simulink model "thrust_control"  (R2017a)
settings: Solver=VariableStepAuto  StartTime=0.0  StopTime=2  MaxStep=1e-3  RelTol=1e-3
values from neighbouring files (symbols this model uses):
  A = [0 1 ... (first row only)    [system_id.m]    (also in thrust_control_data.m)
  Ad = [Ad ... (first row only)    [thrust_control_data.m]
  B = [0 ... (first row only)    [system_id.m]    (also in thrust_control_data.m)
  Bd = [zeros(n+l-1, 1) ... (first row only)    [thrust_control_data.m]
  C = [1 0]    [system_id.m]    (also in thrust_control_data.m)
  Hd = acker(Aobs', Cobs', 0.4 * ones(1, n+l+1))'    [thrust_control_data.m]
  Kd = [2000 1000]    [thrust_control_data.m]
  T = 1/30    (= 0.0333333333333)    [drone_data_process.m]    (also in thrust_control_data.m)
settings Model: Creator=sdc  LastModifiedBy=sdc

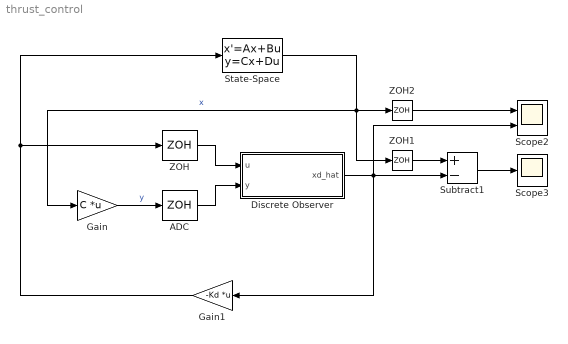
== system thrust_control ==
  ADC : ZeroOrderHold  SampleTime=T
  Discrete Observer : Subsystem
  Gain : Gain  Gain=C  Multiplication=Matrix(K*u)
  Gain1 : Gain  Gain=-Kd  Multiplication=Matrix(K*u)
  Scope2 : Scope  NumInputPorts=2
  Scope3 : Scope
  State-Space : StateSpace  A=A  B=B  C=eye(2)  D=zeros(2,1)  X0=[1;0.1]
  Subtract1 : Sum  Inputs=+-
  ZOH : ZeroOrderHold  SampleTime=T
  ZOH1 : ZeroOrderHold  SampleTime=T
  ZOH2 : ZeroOrderHold  SampleTime=T
  wires:
  Gain1/1 -> State-Space/1, ZOH/1
  State-Space/1 -> ZOH1/1, ZOH2/1, Gain/1  "x"
  Gain/1 -> ADC/1  "y"
  ZOH/1 -> Discrete Observer/1(u)
  ADC/1 -> Discrete Observer/2(y)
  Discrete Observer/1(xd_hat) -> Gain1/1, Subtract1/2, Scope2/2
  Subtract1/1 -> Scope3/1
  ZOH1/1 -> Subtract1/1
  ZOH2/1 -> Scope2/1

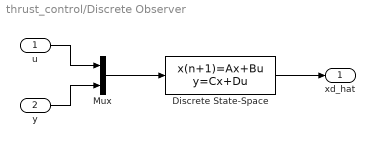
== system thrust_control/Discrete Observer ==
  u : Inport
  y : Inport  Port=2
  Discrete State-Space : DiscreteStateSpace  A=Ad-Hd*C  B=[Bd, Hd]  C=eye(2)  D=zeros(2,2)  SampleTime=T
  Mux : Mux  Inputs=2
  xd_hat : Outport
  wires:
  u/1 -> Mux/1
  y/1 -> Mux/2
  Mux/1 -> Discrete State-Space/1
  Discrete State-Space/1 -> xd_hat/1
